simulink model "motion_gen_unit_test"  (R2025a)
settings: Solver=FixedStepDiscrete  StartTime=0.0  StopTime=5  FixedStep=0.001  RelTol=1e-3  EnableMultiTasking=on
PreLoadFcn:
  | frs = FrankaRobotSettings;
libraries: franka_simulink x1
settings Model: SimulationMode=external  ExtModeTrigDuration=10000  Creator=vasi_ko  LastModifiedBy=kvasios
settings SolverCC: ConcurrentTasks=on  AlgebraicLoopSolver=TrustRegion  InsertRTBMode=Never (minimum delay)
settings DataIOCC: LimitDataPoints=on  SaveFormat=Array  ReturnWorkspaceOutputs=off
settings OptimizationCC: EnhancedBackFolding=on  PassReuseOutputArgsThreshold=0.0  MaxStackSize=200000  OptimizeBlockOrder=speed  DifferentSizesBufferReuse=on  OptimizationCustomize=off
settings DebuggingCC: SolverPrmCheckMsg=warning  ParameterTunabilityLossMsg=error  UnconnectedInputMsg=warning  UnconnectedOutputMsg=warning  UnconnectedLineMsg=warning  SFUnexpectedBacktrackingDiag=warning  SFNoUnconditionalDefaultTransitionDiag=warning  SFExecutionAtInitializationDiag=none  ArithmeticOperatorsInVariantConditions=warning
settings HardwareCC: ProdBitPerLong=64.0  ProdHWDeviceType=Intel->x86-64 (Linux 64)
settings ModelReferenceCC: EnableRefExpFcnMdlSchedulingChecks=on  PropagateSignalLabelsOutOfModel=off
settings SFSimCC: SimUseLocalCustomCode=off  MATLABDynamicMemAlloc=off  CustomCodeUndefinedFunction=UseInterfaceOnly  SimTargetLang=C++  SimDLTargetLibrary=mkl-dnn
settings RTWCC: HardwareBoard=Generic Linux AMD64 Board  RTWVerbose=off  RTWUseLocalCustomCode=off  BuildConfiguration=Faster Runs  TargetLang=C++  GPUComputeCapability=3.5  DLArmComputeVersion=19.05
settings CodeAppCC: ForceParamTrailComments=on  OperatorAnnotations=on
settings GRTTargetCC: ExtMode=on  ExtModeStaticAlloc=on  ExtModeMexFile=ext_xcp  ExtModeIntrfLevel=Level2 - Open  MultiInstanceErrorCode=Warning  TargetLangStandard=C++14 (ISO)
settings ConfigComp: CovMetricSettings=dw  CovSaveCumulativeToWorkspaceVar=on  CovSaveSingleToWorkspaceVar=on  CovExternalEMLEnable=off  CovSFcnEnable=off

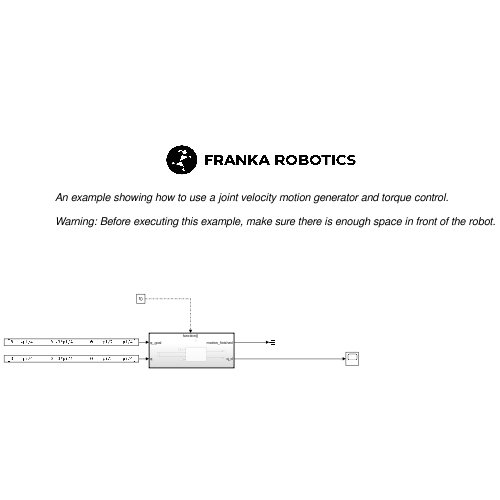
[thumbnail: Simulink's stored preview of the top-level diagram]
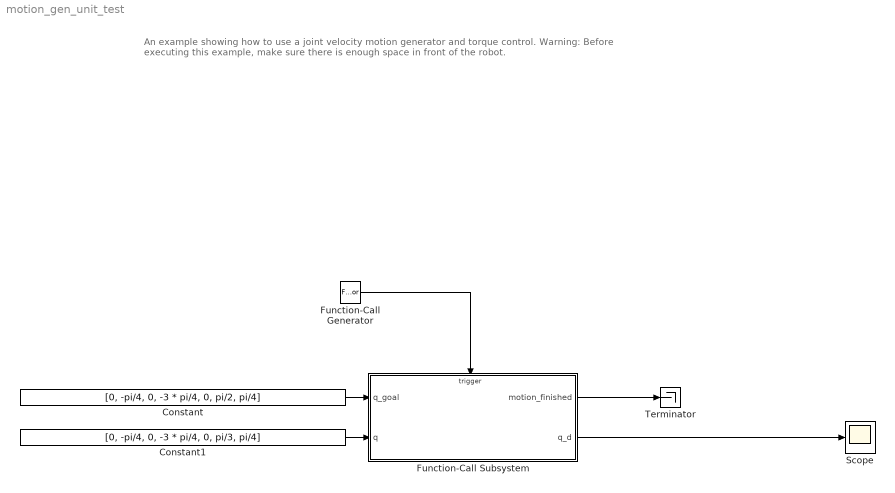
== system motion_gen_unit_test ==
  note: An example showing how to use a joint velocity motion generator and torque control.
      |
      | Warning: Before executing this example, make sure there is enough space in front of the robot.
  Constant : Constant  Value=[0, -pi/4, 0, -3 * pi/4, 0, pi/2, pi/4]
  Constant1 : Constant  Value=[0, -pi/4, 0, -3 * pi/4, 0, pi/3, pi/4]
  Function-Call Generator : FunctionCallGenerator  SampleTime=0.001
  Function-Call Subsystem : Subsystem  TreatAsAtomicUnit=on
      settings: RTWSystemCode=Nonreusable function
  Scope : Scope
      settings: ActiveDisplayYMinimum=-2.8470683423157497  ActiveDisplayYMaximum=2.0616701789183018
  Terminator : Terminator
  wires:
  Function-Call Subsystem/1(motion_finished) -> Terminator/1
  Constant/1 -> Function-Call Subsystem/1(q_goal)
  Constant1/1 -> Function-Call Subsystem/2(q)
  Function-Call Generator/1 -> Function-Call Subsystem/Trigger
  Function-Call Subsystem/2(q_d) -> Scope/1

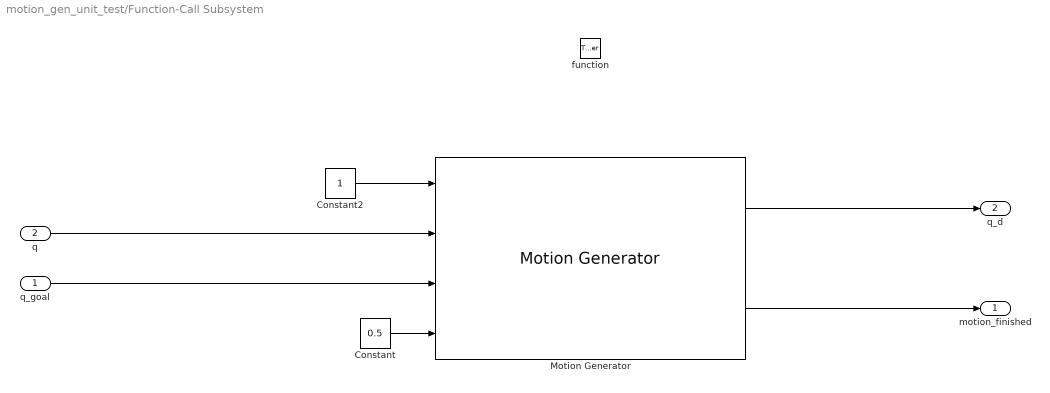
== system motion_gen_unit_test/Function-Call Subsystem ==
  q_goal : Inport
  q : Inport  Port=2
  function : TriggerPort  TriggerType=function-call  VariantControl=(inherit)
  Constant : Constant  Value=0.5
  Constant2 : Constant
  Motion Generator : franka_simulink/Motion Generator
      settings: SourceProductName=Franka Robotics Simulink Support Package
  motion_finished : Outport  InitialOutput=0
  q_d : Outport  Port=2  InitialOutput=zeros(7,1)
  wires:
  Motion Generator/1 -> q_d/1
  Constant/1 -> Motion Generator/4
  q_goal/1 -> Motion Generator/3
  q/1 -> Motion Generator/2
  Constant2/1 -> Motion Generator/1
  Motion Generator/2 -> motion_finished/1
